simulink model "Project_Model_simulink_version_13_6_2023"  (R2021a)
settings: Solver=FixedStepDiscrete  StartTime=0.0  StopTime=10.0  RelTol=1e-3
settings Model: Creator=A  LastModifiedBy=A
settings SolverCC: AlgebraicLoopSolver=TrustRegion

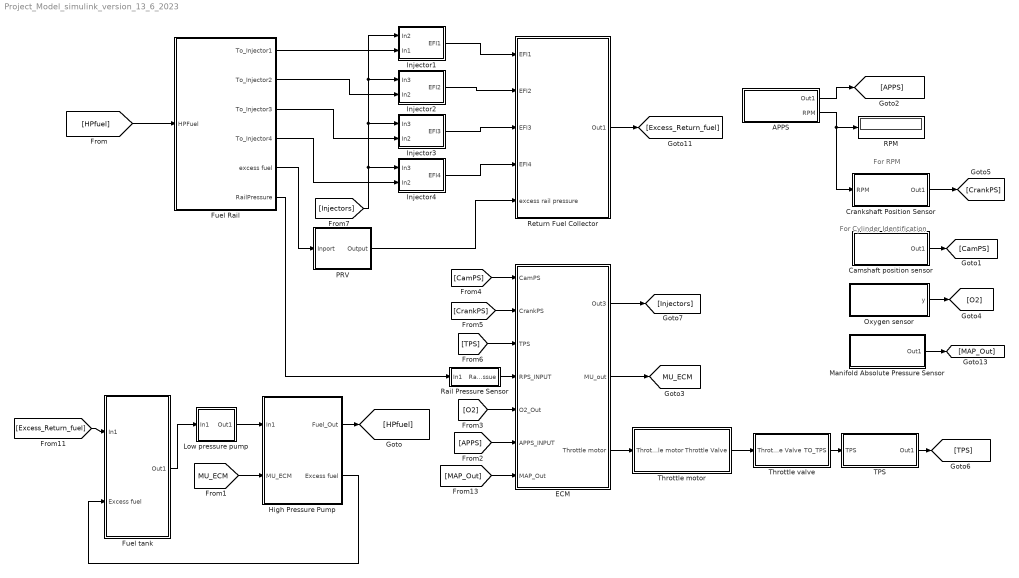
== system Project_Model_simulink_version_13_6_2023 ==
  note: For Cylinder Identification
  note: For RPM
  APPS : Subsystem
  Camshaft position sensor : Subsystem
  Crankshaft Position Sensor : Subsystem
  ECM : Subsystem
  Fuel Rail : Subsystem
  Fuel tank : Subsystem
  High Pressure Pump : Subsystem
  Injector1 : Subsystem
  Injector2 : Subsystem
  Injector3 : Subsystem
  Injector4 : Subsystem
  Low pressure pump : Subsystem
  Manifold Absolute Pressure Sensor : Subsystem
  Oxygen sensor : Subsystem
  PRV : Subsystem
  RPM : Display
  Rail Pressure Sensor : Subsystem
  Return Fuel Collector : Subsystem
  TPS : Subsystem
  Throttle motor : Subsystem
  Throttle valve : Subsystem
  tag scope: MU_ECM=global
  wires:
  Low pressure pump/1(Out1) -> High Pressure Pump/1(In1)
  Fuel tank/1(Out1) -> Low pressure pump/1(In1)
  APPS/1(Out1) -> [APPS]
  [APPS] -> ECM/6(APPS_INPUT)
  ECM/2(MU_out) -> [MU_ECM]
  [O2] -> ECM/5(O2_Out)
  Oxygen sensor/1(y) -> [O2]
  [MU_ECM] -> High Pressure Pump/2(MU_ECM)
  Camshaft position sensor/1(Out1) -> [CamPS]
  Fuel Rail/6(RailPressure) -> Rail Pressure Sensor/1(In1)
  Rail Pressure Sensor/1(Rail Pressue) -> ECM/4(RPS_INPUT)
  [CamPS] -> ECM/1(CamPS)
  [CrankPS] -> ECM/2(CrankPS)
  Crankshaft Position Sensor/1(Out1) -> [CrankPS]
  Injector1/1(EFI1) -> Return Fuel Collector/1(EFI1)
  Injector4/1(EFI4) -> Return Fuel Collector/4(EFI4)
  Injector2/1(EFI2) -> Return Fuel Collector/2(EFI2)
  Injector3/1(EFI3) -> Return Fuel Collector/3(EFI3)
  Fuel Rail/1(To_Injector1) -> Injector1/2(In1)
  Fuel Rail/2(To_Injector2) -> Injector2/2(In2)
  Fuel Rail/3(To_Injector3) -> Injector3/2(In2)
  Fuel Rail/4(To_Injector4) -> Injector4/2(In2)
  ECM/3(Throttle motor) -> Throttle motor/1(Throttle motor)
  Throttle motor/1(Throttle Valve) -> Throttle valve/1(Throtlle Valve)
  [TPS] -> ECM/3(TPS)
  Fuel Rail/5(excess fuel) -> PRV/1(Inport)
  PRV/1(Output) -> Return Fuel Collector/5(excess rail pressure)
  [Injectors] -> Injector4/1(In3), Injector1/1(In2), Injector2/1(In3), Injector3/1(In3)
  ECM/1(Out3) -> [Injectors]
  Return Fuel Collector/1(Out1) -> [Excess_Return_fuel]
  [Excess_Return_fuel] -> Fuel tank/1(In1)
  Throttle valve/1(TO_TPS) -> TPS/1(TPS)
  TPS/1(Out1) -> [TPS]
  [MAP_Out] -> ECM/7(MAP_Out)
  Manifold Absolute Pressure Sensor/1(Out1) -> [MAP_Out]
  High Pressure Pump/2(Excess fuel) -> Fuel tank/2(Excess fuel)
  High Pressure Pump/1(Fuel_Out) -> [HPfuel]
  [HPfuel] -> Fuel Rail/1(HPFuel)
  APPS/2(RPM) -> Crankshaft Position Sensor/1(RPM), RPM/1

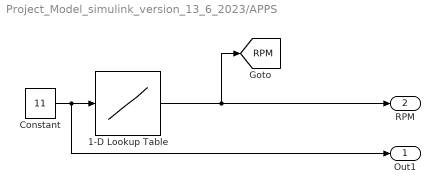
== system Project_Model_simulink_version_13_6_2023/APPS ==
  1-D Lookup Table : Lookup_n-D  NumberOfTableDimensions=1  BreakpointsForDimension1=|  BreakpointsForDimension1DataTypeStr=double  Table=|  TableDataTypeStr=double  ExtrapMethod=Clip  InternalRulePriority=Speed  RndMeth=Simplest  InputSameDT=on
      BreakpointsForDimension1=|
      | [8
      | 10
      | 12
      | 14
      | 16
      | 18
      | 20
      | 22
      | 24
      | 26
      | 28
      | 30
      | 32
      | 34
      | 36
      | 38
      | 40
      | 42
      | 44
      | 46
      | 48
      | 50
      | 52
      | 54
      | 56
      | 58
      | 60
      | 62
      | 64
      | 66
      | 68
      | 70
      | 72
      | 74
      | 76
      | 78
      | 80
      | 82
      | 84
      | 86
      | 88
      | 90]
      Table=|
      | [600
      | 730
      | 860
      | 990
      | 1120
      | 1250
      | 1380
      | 1510
      | 1640
      | 1770
      | 1900
      | 2030
      | 2160
      | 2290
      | 2420
      | 2550
      | 2680
      | 2810
      | 2940
      | 3070
      | 3200
      | 3330
      | 3460
      | 3590
      | 3720
      | 3850
      | 3980
      | 4110
      | 4240
      | 4370
      | 4500
      | 4630
      | 4760
      | 4890
      | 5020
      | 5150
      | 5280
      | 5410
      | 5540
      | 5670
      | 5800
      | 6000]
  Constant : Constant  Value=11
  Out1 : Outport
  RPM : Outport  Port=2
  tag scope: RPM=global
  wires:
  1-D Lookup Table/1 -> [RPM], RPM/1
  Constant/1 -> 1-D Lookup Table/1, Out1/1

== system Project_Model_simulink_version_13_6_2023/Camshaft position sensor ==
  Out1 : Outport
  wires:
  ? -> Out1/1

== system Project_Model_simulink_version_13_6_2023/Crankshaft Position Sensor ==
  RPM : Inport
  Out1 : Outport
  wires:
  RPM/1 -> Out1/1

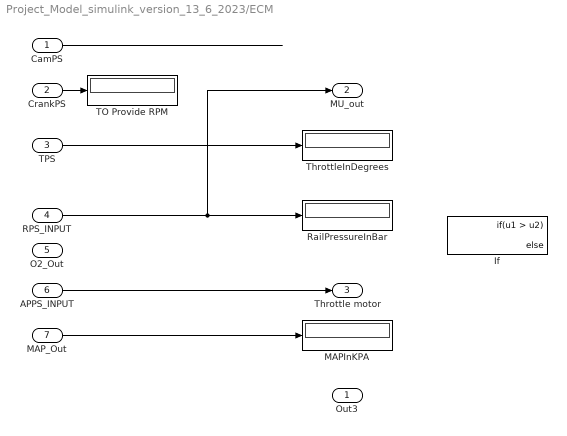
== system Project_Model_simulink_version_13_6_2023/ECM ==
  CamPS : Inport
  CrankPS : Inport  Port=2
  TPS : Inport  Port=3
  RPS_INPUT : Inport  Port=4
  O2_Out : Inport  Port=5
  APPS_INPUT : Inport  Port=6
  MAP_Out : Inport  Port=7
  If : If  NumInputs=2  IfExpression=u1 > u2
  MAPInKPA : Display
  RailPressureInBar : Display
  TO Provide RPM : Display
  ThrottleInDegrees : Display
  Out3 : Outport
  MU_out : Outport  Port=2
  Throttle motor : Outport  Port=3
  wires:
  CamPS/1 -> ?
  APPS_INPUT/1 -> Throttle motor/1
  MAP_Out/1 -> MAPInKPA/1
  TPS/1 -> ThrottleInDegrees/1
  RPS_INPUT/1 -> MU_out/1, RailPressureInBar/1
  CrankPS/1 -> TO Provide RPM/1

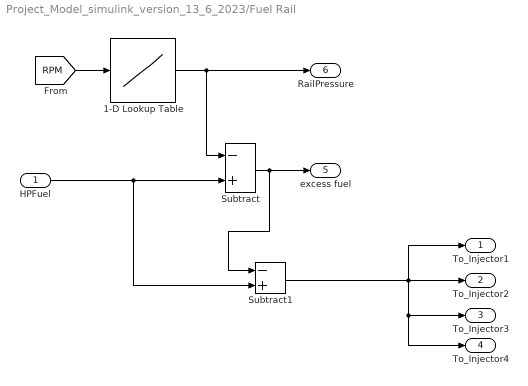
== system Project_Model_simulink_version_13_6_2023/Fuel Rail ==
  HPFuel : Inport
  1-D Lookup Table : Lookup_n-D  NumberOfTableDimensions=1  BreakpointsForDimension1=|  Table=|  InternalRulePriority=Speed  RndMeth=Simplest  InputSameDT=on
      BreakpointsForDimension1=|
      | [600
      | 730
      | 860
      | 990
      | 1120
      | 1250
      | 1380
      | 1510
      | 1640
      | 1770
      | 1900
      | 2030
      | 2160
      | 2290
      | 2420
      | 2550
      | 2680
      | 2810
      | 2940
      | 3070
      | 3200
      | 3330
      | 3460
      | 3590
      | 3720
      | 3850
      | 3980
      | 4110
      | 4240
      | 4370
      | 4500
      | 4630
      | 4760
      | 4890
      | 5020
      | 5150
      | 5280
      | 5410
      | 5540
      | 5670
      | 5800
      | 6000]
      Table=|
      | [300
      | 332
      | 364
      | 396
      | 428
      | 460
      | 492
      | 524
      | 556
      | 588
      | 620
      | 652
      | 684
      | 716
      | 748
      | 780
      | 812
      | 844
      | 876
      | 908
      | 940
      | 972
      | 1004
      | 1036
      | 1068
      | 1100
      | 1132
      | 1164
      | 1196
      | 1228
      | 1260
      | 1292
      | 1324
      | 1356
      | 1388
      | 1420
      | 1452
      | 1484
      | 1516
      | 1548
      | 1580
      | 1600]
  Subtract : Sum  Inputs=-+
  Subtract1 : Sum  Inputs=-+
  To_Injector1 : Outport
  To_Injector2 : Outport  Port=2
  To_Injector3 : Outport  Port=3
  To_Injector4 : Outport  Port=4
  excess fuel : Outport  Port=5
  RailPressure : Outport  Port=6
  wires:
  1-D Lookup Table/1 -> Subtract/1, RailPressure/1
  [RPM] -> 1-D Lookup Table/1
  HPFuel/1 -> Subtract1/2, Subtract/2
  Subtract/1 -> Subtract1/1, excess fuel/1
  Subtract1/1 -> To_Injector1/1, To_Injector4/1, To_Injector3/1, To_Injector2/1

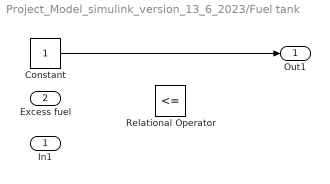
== system Project_Model_simulink_version_13_6_2023/Fuel tank ==
  In1 : Inport
  Excess fuel : Inport  Port=2
  Constant : Constant
  Relational Operator : RelationalOperator  Operator=<=  OutDataTypeStr=boolean  RndMeth=Simplest
  Out1 : Outport
  wires:
  Constant/1 -> Out1/1

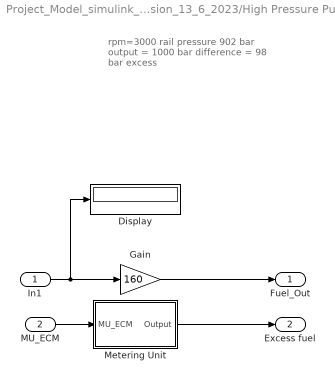
== system Project_Model_simulink_version_13_6_2023/High Pressure Pump ==
  note: rpm=3000
      | rail pressure 902 bar
      | output = 1000 bar
      | difference = 98 bar excess
  In1 : Inport
  MU_ECM : Inport  Port=2
  Display : Display
  Gain : Gain  Gain=160
  Metering Unit : Subsystem
  Fuel_Out : Outport
  Excess fuel : Outport  Port=2
  wires:
  In1/1 -> Gain/1, Display/1
  MU_ECM/1 -> Metering Unit/1(MU_ECM)
  Metering Unit/1(Output) -> Excess fuel/1
  Gain/1 -> Fuel_Out/1

== system Project_Model_simulink_version_13_6_2023/Injector1 ==
  In2 : Inport
  In1 : Inport  Port=2
  EFI1 : Outport
  wires:
  In1/1 -> EFI1/1

== system Project_Model_simulink_version_13_6_2023/Injector2 ==
  In3 : Inport
  In2 : Inport  Port=2
  EFI2 : Outport
  wires:
  ? -> EFI2/1

== system Project_Model_simulink_version_13_6_2023/Injector3 ==
  In3 : Inport
  In2 : Inport  Port=2
  EFI3 : Outport
  wires:
  ? -> EFI3/1

== system Project_Model_simulink_version_13_6_2023/Injector4 ==
  In3 : Inport
  In2 : Inport  Port=2
  EFI4 : Outport
  wires:
  ? -> EFI4/1

== system Project_Model_simulink_version_13_6_2023/Low pressure pump ==
  In1 : Inport
  Gain : Gain  Gain=10
  Out1 : Outport
  wires:
  In1/1 -> Gain/1
  Gain/1 -> Out1/1

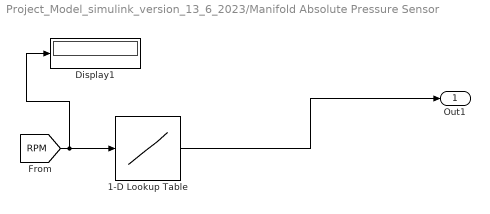
== system Project_Model_simulink_version_13_6_2023/Manifold Absolute Pressure Sensor ==
  1-D Lookup Table : Lookup_n-D  NumberOfTableDimensions=1  BreakpointsForDimension1=|  Table=|  InternalRulePriority=Speed  RndMeth=Simplest  InputSameDT=on
      BreakpointsForDimension1=|
      | [600
      | 730
      | 860
      | 990
      | 1120
      | 1250
      | 1380
      | 1510
      | 1640
      | 1770
      | 1900
      | 2030
      | 2160
      | 2290
      | 2420
      | 2550
      | 2680
      | 2810
      | 2940
      | 3070
      | 3200
      | 3330
      | 3460
      | 3590
      | 3720
      | 3850
      | 3980
      | 4110
      | 4240
      | 4370
      | 4500
      | 4630
      | 4760
      | 4890
      | 5020
      | 5150
      | 5280
      | 5410
      | 5540
      | 5670
      | 5800
      | 6000]
      Table=|
      | [24
      | 24.2
      | 24.3
      | 24.5
      | 24.6
      | 24.8
      | 24.9
      | 25.1
      | 25.2
      | 25.4
      | 25.5
      | 25.7
      | 25.8
      | 26.0
      | 26.1
      | 26.3
      | 26.4
      | 26.6
      | 26.7
      | 26.9
      | 27.0
      | 27.2
      | 27.3
      | 27.5
      | 27.6
      | 27.8
      | 27.9
      | 28.1
      | 28.2
      | 28.4
      | 28.5
      | 28.7
      | 28.8
      | 29.0
      | 29.1
      | 29.3
      | 29.4
      | 29.5
      | 29.7
      | 29.8
      | 29.9
      | 30]
  Display1 : Display
  Out1 : Outport
  wires:
  1-D Lookup Table/1 -> Out1/1
  [RPM] -> Display1/1, 1-D Lookup Table/1

== system Project_Model_simulink_version_13_6_2023/Oxygen sensor ==
  Constant : Constant
  MATLAB Function : MATLAB Function  TreatAsAtomicUnit=on
  y : Outport
  wires:
  MATLAB Function/1(out) -> y/1
  Constant/1 -> MATLAB Function/1(u)

== system Project_Model_simulink_version_13_6_2023/PRV ==
  Inport : Inport
  Output : Outport
  wires:
  Inport/1 -> Output/1

== system Project_Model_simulink_version_13_6_2023/Rail Pressure Sensor ==
  In1 : Inport
  Rail Pressue : Outport
  wires:
  In1/1 -> Rail Pressue/1

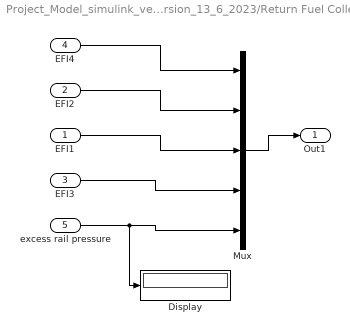
== system Project_Model_simulink_version_13_6_2023/Return Fuel Collector ==
  EFI1 : Inport
  EFI2 : Inport  Port=2
  EFI3 : Inport  Port=3
  EFI4 : Inport  Port=4
  excess rail pressure : Inport  Port=5
  Display : Display
  Mux : Mux  Inputs=5
  Out1 : Outport
  wires:
  EFI4/1 -> Mux/1
  EFI2/1 -> Mux/2
  EFI1/1 -> Mux/3
  EFI3/1 -> Mux/4
  excess rail pressure/1 -> Display/1, Mux/5
  Mux/1 -> Out1/1

== system Project_Model_simulink_version_13_6_2023/TPS ==
  TPS : Inport
  Out1 : Outport
  wires:
  TPS/1 -> Out1/1

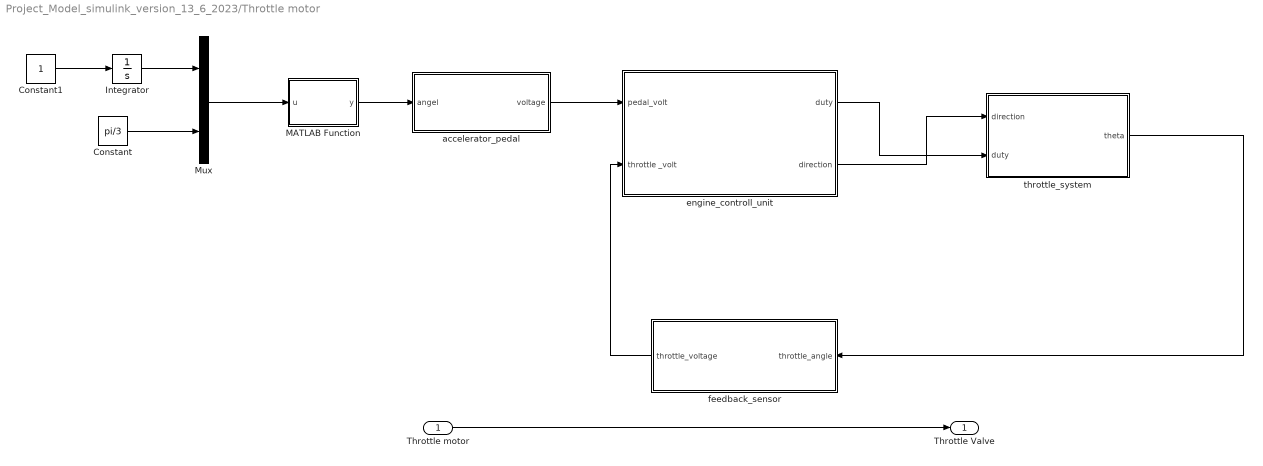
== system Project_Model_simulink_version_13_6_2023/Throttle motor ==
  Throttle motor : Inport
  Constant : Constant  Value=pi/3
  Constant1 : Constant
  Integrator : Integrator
  MATLAB Function : MATLAB Function  TreatAsAtomicUnit=on
  Mux : Mux  Inputs=2
  accelerator_pedal : Subsystem
  engine_controll_unit : Subsystem
  feedback_sensor : Subsystem
      settings: PortSchema="{\"entries\":[{\"content\":{\"sides\":[{\"content\":{\"connectorIds\":[\"Out1\"]},\"type\":\"ConnectorPlacement.EquallySpacedRectSide\",\"uuid\":\"fe640009-eb11-44be-8596-49d62a5beec8\"},{\"content\":{\"connectorIds\":[\"In1\"],\"side\":\"RIGHT\"},\"type\":\"ConnectorPlacement.EquallySpacedRectSide\",\"uuid\":\"55096441-78fe-4501-a0f7-12f27b21a046\"},{\"content\":{\"connectorIds\":[],\"side\":\"TOP\"},\"type\":\"ConnectorPlacement.EquallySpacedRectSide\",\"uuid\":\"eb36a32d-1c61-4111-82c5-835a656f9bf6\"}]},\"type\":\"ConnectorPlacement.EquallySpacedConnector\",\"uuid\":\"24611814-9bea-49d8-8ce5-1a9dc2d12b43\"}],\"packageUris\":[\"http://schema.mathworks.com/mf0/Connector/R2020b\"],\"version\":\"1.0\"}"
  throttle_system : Subsystem
  Throttle Valve : Outport
  wires:
  Throttle motor/1 -> Throttle Valve/1
  MATLAB Function/1(y) -> accelerator_pedal/1(angel)
  Mux/1 -> MATLAB Function/1(u)
  engine_controll_unit/1(duty) -> throttle_system/2(duty)
  throttle_system/1(theta) -> feedback_sensor/1(throttle_angle)
  engine_controll_unit/2(direction) -> throttle_system/1(direction)
  Constant1/1 -> Integrator/1
  accelerator_pedal/1(voltage) -> engine_controll_unit/1(pedal_volt)
  feedback_sensor/1(throttle_voltage) -> engine_controll_unit/2(throttle _volt)
  Integrator/1 -> Mux/1
  Constant/1 -> Mux/2

== system Project_Model_simulink_version_13_6_2023/Throttle valve ==
  Throtlle Valve : Inport
  TO_TPS : Outport
  wires:
  Throtlle Valve/1 -> TO_TPS/1

== system Project_Model_simulink_version_13_6_2023/High Pressure Pump/Metering Unit ==
  note: if fuel pressure in rail is as per the required in specific rpm then duty cycle is 15 % if pressure is more duty cylce will increase to 20 % until pressure in rail is as per required
  MU_ECM : Inport
  Output : Outport
  wires:
  MU_ECM/1 -> Output/1

== system Project_Model_simulink_version_13_6_2023/Throttle motor/accelerator_pedal ==
  angel : Inport
  1-D Lookup Table : Lookup_n-D  NumberOfTableDimensions=1  BreakpointsForDimension1=[0 90]  Table=[0.5 4.5]  InternalRulePriority=Speed  RndMeth=Simplest  InputSameDT=on
  Gain : Gain  Gain=180/pi
  voltage : Outport
  wires:
  1-D Lookup Table/1 -> voltage/1
  Gain/1 -> 1-D Lookup Table/1
  angel/1 -> Gain/1

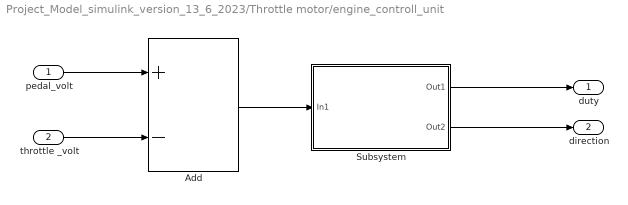
== system Project_Model_simulink_version_13_6_2023/Throttle motor/engine_controll_unit ==
  pedal_volt : Inport
  throttle _volt : Inport  Port=2
  Add : Sum  Inputs=+-
  Subsystem : Subsystem
  duty : Outport
  direction : Outport  Port=2
  wires:
  Add/1 -> Subsystem/1(In1)
  pedal_volt/1 -> Add/1
  throttle _volt/1 -> Add/2
  Subsystem/1(Out1) -> duty/1
  Subsystem/2(Out2) -> direction/1

== system Project_Model_simulink_version_13_6_2023/Throttle motor/feedback_sensor ==
  throttle_angle : Inport
  Subsystem : Subsystem
  throttle_voltage : Outport
  wires:
  throttle_angle/1 -> Subsystem/1(angle)
  Subsystem/1(voltage) -> throttle_voltage/1

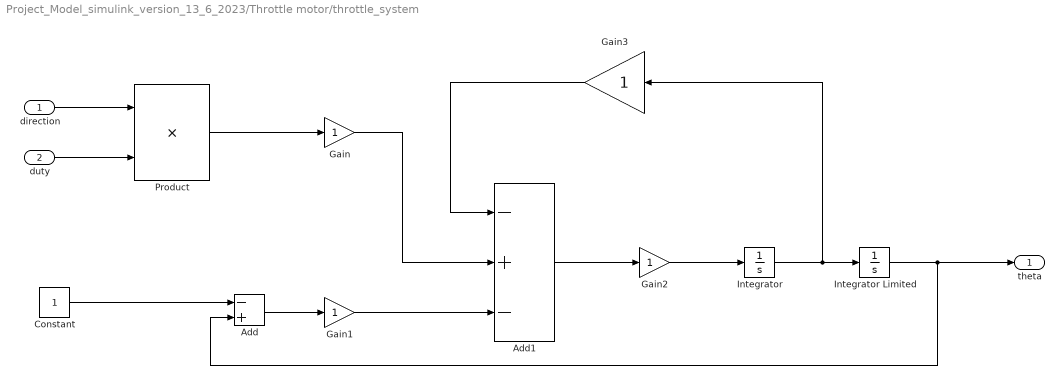
== system Project_Model_simulink_version_13_6_2023/Throttle motor/throttle_system ==
  direction : Inport
  duty : Inport  Port=2
  Add : Sum  Inputs=-+
  Add1 : Sum  Inputs=-+-
  Constant : Constant
  Gain{,1..3} (4 alike) : Gain
  Integrator : Integrator
  Integrator Limited : Integrator  LimitOutput=on  UpperSaturationLimit=pi/2  LowerSaturationLimit=0
  Product : Product
  theta : Outport
  wires:
  direction/1 -> Product/1
  duty/1 -> Product/2
  Product/1 -> Gain/1
  Add/1 -> Gain1/1
  Gain/1 -> Add1/2
  Gain1/1 -> Add1/3
  Constant/1 -> Add/1
  Gain2/1 -> Integrator/1
  Add1/1 -> Gain2/1
  Integrator/1 -> Gain3/1, Integrator Limited/1
  Integrator Limited/1 -> Add/2, theta/1
  Gain3/1 -> Add1/1

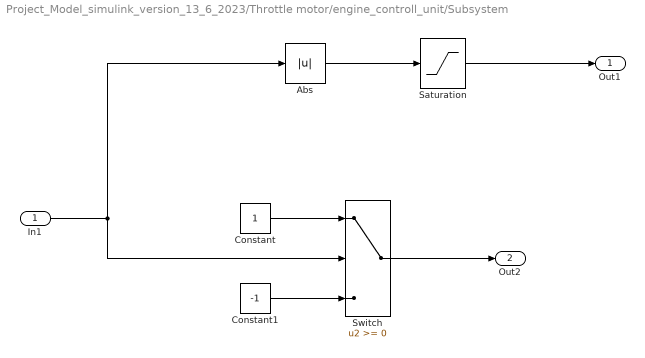
== system Project_Model_simulink_version_13_6_2023/Throttle motor/engine_controll_unit/Subsystem ==
  In1 : Inport
  Abs : Abs
  Constant : Constant
  Constant1 : Constant  Value=-1
  Saturation : Saturate
  Switch : Switch
  Out1 : Outport
  Out2 : Outport  Port=2
  wires:
  Abs/1 -> Saturation/1
  In1/1 -> Switch/2, Abs/1
  Constant/1 -> Switch/1
  Constant1/1 -> Switch/3
  Saturation/1 -> Out1/1
  Switch/1 -> Out2/1

== system Project_Model_simulink_version_13_6_2023/Throttle motor/feedback_sensor/Subsystem ==
  angle : Inport
  1-D Lookup Table : Lookup_n-D  NumberOfTableDimensions=1  BreakpointsForDimension1=[0 90]  Table=[0.5 4.5]  InternalRulePriority=Speed  RndMeth=Simplest  InputSameDT=on
  Gain : Gain  Gain=180/pi
  voltage : Outport
  wires:
  1-D Lookup Table/1 -> voltage/1
  Gain/1 -> 1-D Lookup Table/1
  angle/1 -> Gain/1

== matlab function Project_Model_simulink_version_13_6_2023/Oxygen sensor/MATLAB Function ==
  data: u input; out output
function out = fcn(u)
%#codegen

if (u>0.65)
y = 0.95;
elseif (u<=0.65 && u>=0.25)
    y = 1;
else
    y=1.05;
end

out=y;

== matlab function Project_Model_simulink_version_13_6_2023/Throttle motor/MATLAB Function ==
  data: u input; y output
function y = fcn(u)

y = u;
